simulink model "sfcndemo_mixedm"  (Simulink 6.0)
settings: Solver=ode5  SolverMode=SingleTasking  StartTime=0.0  StopTime=10.0  FixedStep=.1  MaxStep=.1  RelTol=1e-3  AbsTol=1e-6
settings Model: Creator=The MathWorks Inc.  LastModifiedBy=batserve  ExtModeTrigMode=oneshot  ExtModeArmWhenConnect=off  ExtModeAutoUpdateStatusClock=off
settings DataIOCC: ExternalInput=[]  InitialState=[]  LimitDataPoints=off  TimeSaveName=t  OutputSaveName=y
settings OptimizationCC: BooleanDataType=off
settings DebuggingCC: CheckExecutionContextPreStartOutputMsg=on  CheckExecutionContextRuntimeOutputMsg=on  SolverPrmCheckMsg=none  InheritedTsInSrcMsg=none  IntegerOverflowMsg=none
settings HardwareCC: TargetUnknown=on

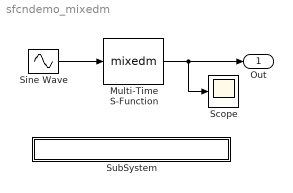
== system sfcndemo_mixedm ==
  Multi-Time S-Function : S-Function  FunctionName=mixedm
      mask Type: S-function: mixedm
      mask Description: This is a S-function that illustrates multiple sample time by implementing integrator -> ZOH(Ts=1second) -> UnitDelay(Ts=1second) with an initial condition of 1.
  Scope : Scope
      settings: TimeRange=10  YMin=1  YMax=3
  Sine Wave : Sin  SampleTime=0
  SubSystem : Subsystem  PropExecContextAcrossSSBoundary=on
      settings: OpenFcn=edit(fullfile(matlabroot,'simulink','src','mixedm.c'))
      mask Display: disp('matlabroot\simulink\src\mixedm.c');
  Out : Outport  InitialOutput=0
  wires:
  Sine Wave/1 -> Multi-Time S-Function/1
  Multi-Time S-Function/1 -> Out/1, Scope/1

== system sfcndemo_mixedm/SubSystem ==
